simulink model "practica13_2017a"  (R2017a)
settings: Solver=VariableStepAuto  StartTime=0.0  StopTime=100  RelTol=1e-3
values from neighbouring files (symbols this model uses):
  A_1 = 1    [Practica 1.3.m]    (also in practica1Parte2.m)
  a_1 = 0.1    [Practica 1.3.m]    (also in practica1Parte2.m)
  A_2 = 1    [Practica 1.3.m]    (also in practica1Parte2.m)
  a_2 = 0.1    [Practica 1.3.m]    (also in practica1Parte2.m)
  g = 9.81    [Practica 1.3.m]    (also in pactica1.m = 9.8; practica1Parte2.m)
  gamma = 0.6    [Practica 1.3.m]    (also in practica1Parte2.m)
  Ts = 0.001    [Practica 1.3.m]
libraries: simulink x1
settings Model: Creator=Andres Zambrano  LastModifiedBy=af.zambrano82

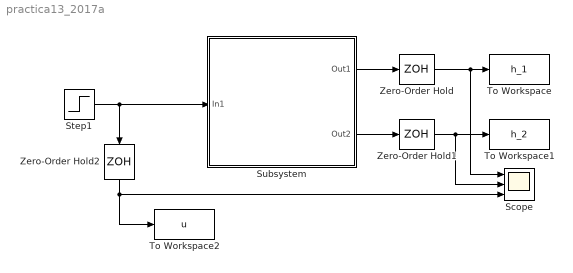
== system practica13_2017a ==
  Scope : Scope  NumInputPorts=3
  Step1 : Step  SampleTime=0
  Subsystem : Subsystem
  To Workspace : ToWorkspace  VariableName=h_1  SampleTime=-1
      settings: Save2DSignal=2-D array (concatenate along first dimension)
  To Workspace1 : ToWorkspace  VariableName=h_2  SampleTime=-1
      settings: Save2DSignal=2-D array (concatenate along first dimension)
  To Workspace2 : ToWorkspace  VariableName=u  SampleTime=-1
      settings: Save2DSignal=2-D array (concatenate along first dimension)
  Zero-Order Hold : ZeroOrderHold  SampleTime=Ts
  Zero-Order Hold1 : ZeroOrderHold  SampleTime=Ts
  Zero-Order Hold2 : ZeroOrderHold  SampleTime=Ts
  wires:
  Zero-Order Hold/1 -> Scope/1, To Workspace/1
  Zero-Order Hold1/1 -> Scope/2, To Workspace1/1
  Subsystem/2(Out2) -> Zero-Order Hold1/1
  Zero-Order Hold2/1 -> To Workspace2/1, Scope/3
  Subsystem/1(Out1) -> Zero-Order Hold/1
  Step1/1 -> Subsystem/1(In1), Zero-Order Hold2/1

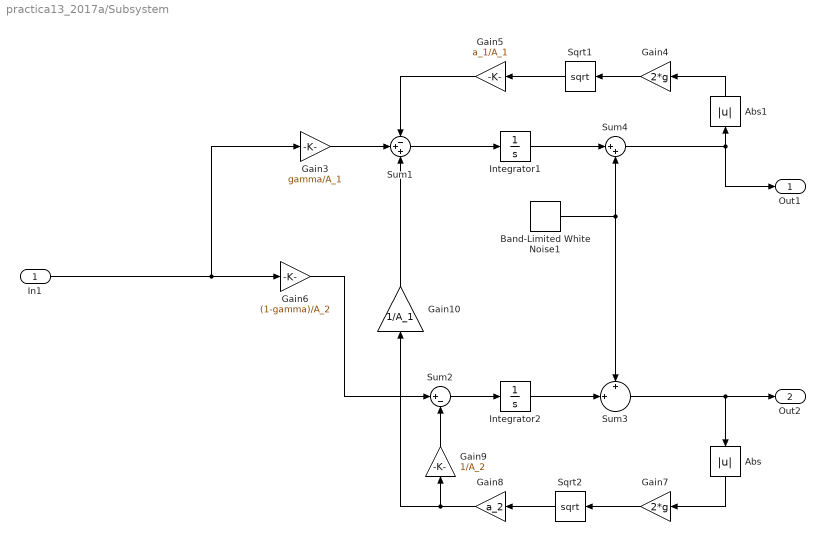
== system practica13_2017a/Subsystem ==
  In1 : Inport
  Abs : Abs
  Abs1 : Abs
  Band-Limited White Noise1 : simulink/Sources/Band-Limited White Noise  Cov=[1e-4]  Ts=0.1  seed=[23341]
  Gain10 : Gain  Gain=1/A_1
  Gain3 : Gain  Gain=gamma/A_1
  Gain4 : Gain  Gain=2*g
  Gain5 : Gain  Gain=a_1/A_1
  Gain6 : Gain  Gain=(1-gamma)/A_2
  Gain7 : Gain  Gain=2*g
  Gain8 : Gain  Gain=a_2
  Gain9 : Gain  Gain=1/A_2
  Integrator1 : Integrator
  Integrator2 : Integrator
  Sqrt1 : Sqrt  SaturateOnIntegerOverflow=on
  Sqrt2 : Sqrt  SaturateOnIntegerOverflow=on
  Sum1 : Sum  Inputs=-++
  Sum2 : Sum  Inputs=|+-
  Sum3 : Sum  Inputs=+|+||
  Sum4 : Sum  Inputs=|++
  Out1 : Outport
  Out2 : Outport  Port=2
  wires:
  Integrator2/1 -> Sum3/2
  Gain8/1 -> Gain10/1, Gain9/1
  Sqrt2/1 -> Gain8/1
  Gain9/1 -> Sum2/2
  Gain6/1 -> Sum2/1
  Sqrt1/1 -> Gain5/1
  Sum2/1 -> Integrator2/1
  Sum3/1 -> Out2/1, Abs/1
  Gain10/1 -> Sum1/3
  Band-Limited White Noise1/1 -> Sum3/1, Sum4/2
  Abs/1 -> Gain7/1
  Sum4/1 -> Out1/1, Abs1/1
  Gain5/1 -> Sum1/1
  Gain4/1 -> Sqrt1/1
  Gain7/1 -> Sqrt2/1
  Abs1/1 -> Gain4/1
  Integrator1/1 -> Sum4/1
  Sum1/1 -> Integrator1/1
  In1/1 -> Gain6/1, Gain3/1
  Gain3/1 -> Sum1/2
